simulink model "millingSim"  (R2023a)
settings: Solver=FixedStepDiscrete  StartTime=0.0  StopTime=10.0  RelTol=1e-3
InitFcn:
  | % STEP 1: Initialize model parameters
  | % In Simulink, these become tunable parameters or a Bus for parameter data.
  | initMillingParameters;
  | 
  | % STEP 2: Initialize states
  | % In Simulink, these might become discrete states or Data Store Memory.
  | initMillingStates;
  | 
  | % STEP 3: Pre-allocate storage for logging (optional in Simulink).
  | % logger = initLogger(params);
  | 
  | 
  | %--- Now set the Data Store Memory block's initial value
  | %    Replace 'MillingSimulinkModel' with the *actual* name of your model
  | %    Replace 'StatesDataStore' if you gave the memory block a different name
  | % set_param('millingSim/States Memory', ...
  | %           'InitialValue', 'states');
  | % states_bus = Simulink.Bus.createObject(states);
  | 
  | 
  | % % Create Params Bus for Simulink Model
  | % params_bus_info = Simulink.Bus.createObject(params);
  | % params_bus = evalin('base', params_bus_info.busName);
values from neighbouring files (symbols this model uses):
  Nt = 3    [initMillingParameters.m]    (also in m10_milling.m; m11_milling_CSSV.m; m12_milling_FFT.m; m13_milling_RK4.m)
  params = initMillingParameters()    [m20_milling_simulink.m]
  states = integrateDynamics(states, Fx, Fy, params)    [m20_milling_simulink.m]
  steps_rev = steps_tooth * Nt    [initMillingParameters.m]    (also in m10_milling.m; m11_milling_CSSV.m; m12_milling_FFT.m; m13_milling_RK4.m)
  teeth = zeros(1, Nt)    [initMillingStates.m]    (also in m10_milling.m; m11_milling_CSSV.m; m12_milling_FFT.m; m13_milling_RK4.m)
settings Model: Creator=zhuzhen  LastModifiedBy=zhuzhen

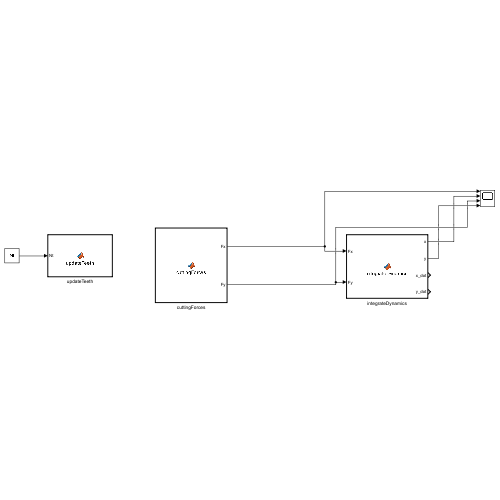
[thumbnail: Simulink's stored preview of the top-level diagram]
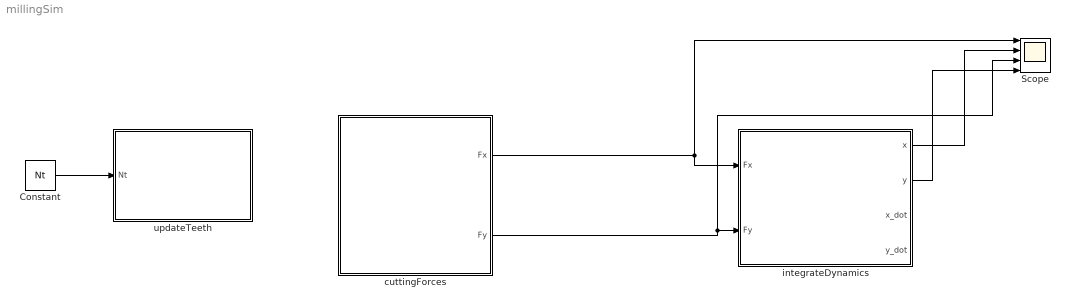
== system millingSim ==
  Constant : Constant  Value=Nt
  Scope : Scope  NumInputPorts=4
  cuttingForces : MATLAB Function  TreatAsAtomicUnit=on
  integrateDynamics : MATLAB Function  TreatAsAtomicUnit=on
  updateTeeth : MATLAB Function  TreatAsAtomicUnit=on
  wires:
  cuttingForces/1(Fx) -> Scope/1, integrateDynamics/1(Fx)
  cuttingForces/2(Fy) -> Scope/3, integrateDynamics/2(Fy)
  integrateDynamics/1(x) -> Scope/2
  integrateDynamics/2(y) -> Scope/4
  Constant/1 -> updateTeeth/1(Nt)

== matlab function millingSim/integrateDynamics ==
  data: Fx input; Fy input; x output; y output; x_dot output; y_dot output; states parameter; params parameter
% Subfunction to integrate structural dynamics
% Could be a MATLAB Function block or System object with discrete states.
function [x, y, x_dot, y_dot] = integrateDynamics(Fx, Fy, states, params)

    % x direction integration
    ddp       = (Fx - params.cx*states.dp - params.kx*states.p) / params.mx;
    states.dp = states.dp + ddp * params.dt;
    states.x_dot = states.dp;  % velocity contribution
    states.p  = states.p + states.dp * params.dt;
    states.x  = states.p;      % total x displacement

    % y direction integration
    ddq       = (Fy - params.cy*states.dq - params.ky*states.q) / params.my;
    states.dq = states.dq + ddq * params.dt;
    states.y_dot = states.dq;  % velocity contribution
    states.q  = states.q + states.dq * params.dt;
    states.y  = states.q;      % total y displacement

    x = states.x;
    y = states.y;
    x_dot = states.x_dot;
    y_dot = states.y_dot;

end

== matlab function millingSim/cuttingForces ==
  data: Fx output; Fy output; params parameter; states parameter
function [Fx, Fy] = cuttingForces(...
    params, states)

    Fx = 0;
    Fy = 0;
    updatedSurf = states.surf;  % local copy to update

    % Expand x, y, x_dot, y_dot for readability
    x     = states.x;
    y     = states.y;
    x_dot = states.x_dot;
    y_dot = states.y_dot;

    for cnt3 = 1:params.Nt
        for cnt4 = 1:params.steps_axial
            phi_counter = states.teeth(cnt3) - (cnt4 - 1);
            if phi_counter < 1
                phi_counter = phi_counter + params.steps_rev;
            end

            phia = params.phi(phi_counter);  % deg

            if (phia >= params.phis) && (phia <= params.phie)
                n      = x*sin(phia*pi/180) - y*cos(phia*pi/180);
                n_dot  = x_dot*sin(phia*pi/180) - y_dot*cos(phia*pi/180);
                h      = params.ft*sin(phia*pi/180) + updatedSurf(cnt4, phi_counter) - n;
                if h < 0
                    Ft = 0;
                    Fn = 0;
                    updatedSurf(cnt4, phi_counter) = ...
                        updatedSurf(cnt4, phi_counter) + params.ft*sin(phia*pi/180);
                else
                    Ft = params.kt * h * axialDiskHeight(params, phia);
                    Fn = params.kn * h * axialDiskHeight(params, phia) ...
                         - params.C * axialDiskHeight(params, phia) ...
                         * (1/params.v) * n_dot;
                    updatedSurf(cnt4, phi_counter) = n;
                end
            else
                Ft = 0;
                Fn = 0;
            end

            Fx = Fx + Ft*cos(phia*pi/180) + Fn*sin(phia*pi/180);
            Fy = Fy + Ft*sin(phia*pi/180) - Fn*cos(phia*pi/180);
        end
    end

    % Write the updated surf back into the output states
    states.surf = updatedSurf;
    states_out = states;
end

% Helper to compute axial disk height (db) as a function of helix, etc.
% In your original code, db is constant along the axial steps,
% but this function might be extended for variable helix.
function db_val = axialDiskHeight(params, ~)
    if params.gamma == 0
        db_val = params.b;
    else
        db_val = params.d * (params.dphi*pi/180) / (2 * tan(params.gamma*pi/180));
    end
end

== matlab function millingSim/updateTeeth ==
  data: teeth parameter; steps_rev parameter; Nt input
% Subfunction to update tooth angles
% In Simulink, this might be part of the main step or a separate subsystem.
function updateTeeth(teeth, steps_rev, Nt)
    for cnt2 = 1:Nt
        teeth(cnt2) = teeth(cnt2) + 1;
        if teeth(cnt2) > steps_rev
            teeth(cnt2) = 1;
        end
    end
end
